simulink model "waterTankControl_sim"  (R2024a)
settings: Solver=VariableStepAuto  StartTime=0.0  StopTime=t_sim  RelTol=1e-3
undefined symbols (not defined in the file): a, g
settings Model: Creator=lorenzo  LastModifiedBy=lorenzo

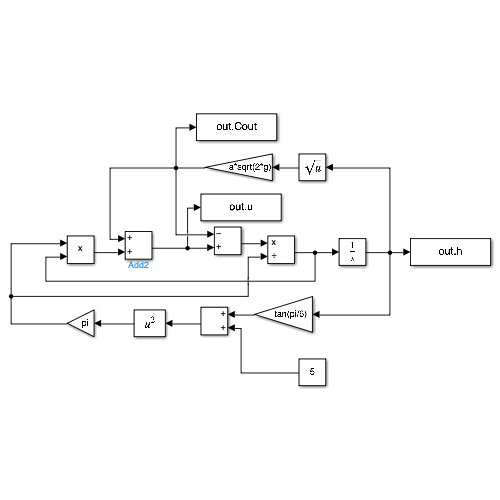
[thumbnail: Simulink's stored preview of the top-level diagram]
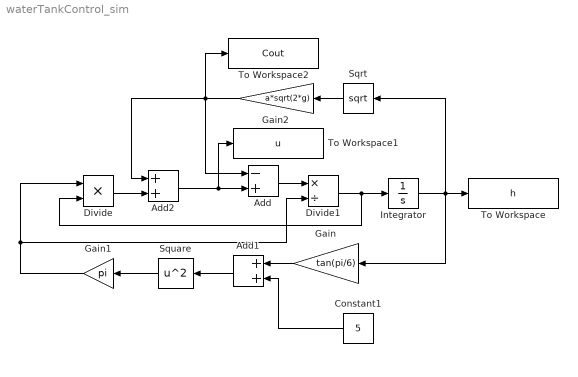
== system waterTankControl_sim ==
  Add : Sum  Inputs=-+
  Add1 : Sum
  Add2 : Sum
  Constant1 : Constant  Value=5
  Divide : Product  Inputs=**
  Divide1 : Product  Inputs=*/
  Gain : Gain  Gain=tan(pi/6)
  Gain1 : Gain  Gain=pi
  Gain2 : Gain  Gain=a*sqrt(2*g)
  Integrator : Integrator  InitialCondition=8
  Sqrt : Sqrt
  Square : Math  Operator=square
  To Workspace : ToWorkspace  VariableName=h  SaveFormat=Timeseries  SampleTime=-1
  To Workspace1 : ToWorkspace  VariableName=u  SaveFormat=Timeseries  SampleTime=-1
  To Workspace2 : ToWorkspace  VariableName=Cout  SaveFormat=Timeseries  SampleTime=-1
  wires:
  Integrator/1 -> Sqrt/1, To Workspace/1, Gain/1
  Square/1 -> Gain1/1
  Gain/1 -> Add1/1
  Add1/1 -> Square/1
  Constant1/1 -> Add1/2
  Sqrt/1 -> Gain2/1
  Gain2/1 -> To Workspace2/1, Add/1, Add2/1
  Gain1/1 -> Divide/1, Divide1/2
  Divide/1 -> Add2/2
  Add2/1 -> To Workspace1/1, Add/2
  Add/1 -> Divide1/1
  Divide1/1 -> Divide/2, Integrator/1
